simulink model "VSC_GFo_Variable_Frequency_v1"  (R2019b)
settings: Solver=ode1  StartTime=0.0  StopTime=8  FixedStep=Time_Step  MaxStep=1e-5  RelTol=1e-3
undefined symbols (not defined in the file): fb, fn, GRD00_H, GRD00_Lg, GRD00_R, GRD00_Rg, GRD00_TD, GRD00_TN, GRD00_Ub, Time_Step, VSC01_id0, VSC01_Lt_pu, VSC01_mp1, VSC01_mp2, VSC01_mp3, VSC01_Pn, VSC01_R, VSC01_Rt_pu, VSC01_Rv, VSC01_Sn, VSC01_T1, VSC01_T2, VSC01_Tr_PLL, VSC01_Udc_n, VSC01_Udcb, VSC01_Un1, VSC01_Un2, VSC01_W_LF, VSC01_wc1, VSC01_wc2, VSC01_wc3
libraries: powerlib x24, powerlib_meascontrol x1
(part 1 of 2)
settings Model: Creator=Frederic_Colas  LastModifiedBy=xguillau
settings DataIOCC: ReturnWorkspaceOutputs=off
settings OptimizationCC: LifeSpan=inf
settings DebuggingCC: UnconnectedInputMsg=none  UnconnectedOutputMsg=none  UnconnectedLineMsg=none  SFExecutionAtInitializationDiag=none  ArithmeticOperatorsInVariantConditions=warning
settings HardwareCC: ProdBitPerSizeT=32  ProdBitPerPtrDiffT=32  ProdWordSize=32  ProdHWDeviceType=Specified
settings SFSimCC: SimUseLocalCustomCode=off  CustomCodeUndefinedFunction=UseInterfaceOnly
settings RTWCC: RTWUseLocalCustomCode=off
settings CodeAppCC: StateflowObjectComments=on
settings SimscapeCC: SimscapeNormalizeSystem=off

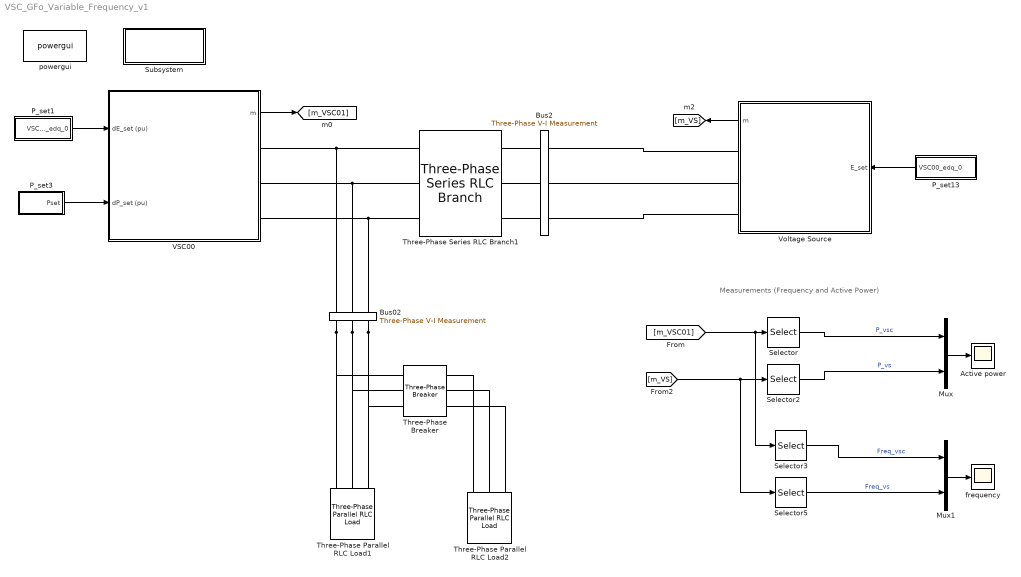
== system VSC_GFo_Variable_Frequency_v1 ==
  note: Measurements (Frequency and Active Power)
  Active power : Scope
  "Bus02 " : powerlib/Measurements/Three-Phase V-I Measurement  VoltageMeasurement=no  SetLabelV=off  LabelV=Vabc  Vpu=off  VpuLL=off  CurrentMeasurement=no  SetLabelI=off  LabelI=Iabc  Ipu=off  Pbase=100e6  Vbase=500e3  OutputType=Complex  PhasorSimulation=off  PSBequivalent=0
      settings: SourceProductName=Simscape Electrical
  Bus2 : powerlib/Measurements/Three-Phase V-I Measurement  VoltageMeasurement=no  SetLabelV=off  LabelV=Vabc  Vpu=off  VpuLL=off  CurrentMeasurement=no  SetLabelI=off  LabelI=Iabc  Ipu=off  Pbase=1e9  Vbase=VSC01_Un2  OutputType=Complex  PhasorSimulation=off  PSBequivalent=0
      settings: SourceProductName=Simscape Electrical
  Mux : Mux  Inputs=2
  Mux1 : Mux  Inputs=2
  P_set1 : Subsystem
  P_set13 : Subsystem
  P_set3 : Subsystem
  Selector : Selector  InputPortWidth=3  IndexOptions=Index vector (dialog)  Indices=[1]  OutputSizes=1
  Selector2 : Selector  InputPortWidth=2  IndexOptions=Index vector (dialog)  Indices=[1]  OutputSizes=1
  Selector3 : Selector  InputPortWidth=3  IndexOptions=Index vector (dialog)  Indices=3  OutputSizes=1
  Selector5 : Selector  InputPortWidth=2  IndexOptions=Index vector (dialog)  Indices=2  OutputSizes=1
  Subsystem : Subsystem
      settings: OpenFcn=LoadFlow_VSC
      mask Display: color('blue'),disp('Update Loadflow')
  Three-Phase Parallel RLC Load1 : powerlib/Elements/Three-Phase Parallel RLC Load  LConnTagsString=A|B|C  Configuration=Y (grounded)  NominalVoltage=GRD00_Un  Vabc=[1e3 1e3 1e3]  Vabcp=[1e3 1e3 1e3]  NominalFrequency=fb  UnbalancedPower=off  ActivePower=100e6  InductivePower=0  CapacitivePower=0  Pabc=[10e3 9e3 11e3]  QLabc=[100 90 110]  QCabc=[100 90 110]  Pabcp=[10e3 9e3 11e3]  QLabcp=[100 90 110]  QCabcp=[100 90 110]  Measurements=None  LoadType=constant Z
      settings: SourceProductName=Simscape Electrical
  Three-Phase Parallel RLC Load2 : powerlib/Elements/Three-Phase Parallel RLC Load  LConnTagsString=A|B|C  Configuration=Y (grounded)  NominalVoltage=GRD00_Un  Vabc=[1e3 1e3 1e3]  Vabcp=[1e3 1e3 1e3]  NominalFrequency=fb  UnbalancedPower=off  ActivePower=400e6  InductivePower=0  CapacitivePower=0  Pabc=[10e3 9e3 11e3]  QLabc=[100 90 110]  QCabc=[100 90 110]  Pabcp=[10e3 9e3 11e3]  QLabcp=[100 90 110]  QCabcp=[100 90 110]  Measurements=None  LoadType=constant Z
      settings: SourceProductName=Simscape Electrical
  Three-Phase Series RLC Branch1 : powerlib/Elements/Three-Phase Series RLC Branch  LConnTagsString=A|B|C  RConnTagsString=A|B|C  BranchType=RL  Resistance=GRD00_Rg  Inductance=GRD00_Lg  Capacitance=1e-6  Measurements=None
      settings: SourceProductName=Simscape Electrical
  Three-Phase Breaker : powerlib/Elements/Three-Phase Breaker  InitialState=open  SwitchA=on  SwitchB=on  SwitchC=on  SwitchTimes=[1 60]  External=off  BreakerResistance=0.01  SnubberResistance=1e6  SnubberCapacitance=inf  Measurements=None
      settings: SourceProductName=Simscape Electrical
  VSC00 : Subsystem  mask(VSC){fb=fb, Sn=VSC01_Sn, Pn=VSC01_Pn, Un1=VSC01_Un1, Un2=VSC01_Un2, Rt_pu=VSC01_Rt_pu, Lt_pu=VSC01_Lt_pu, Lm_pu=500, Rm_pu=500, Tr_PLL=VSC01_Tr_PLL, Val_Freq_Support=on, R_percent=VSC01_R, Rv=VSC01_Rv, W_TVR=VSC01_W_LF, gainpopup=1, wc1=VSC01_wc1, mp1=VSC01_mp1, wc2=VSC01_wc2, mp2=VSC01_mp2, wc3=VSC01_wc3, mp3=VSC01_mp3, T1=VSC01_T1, T2=VSC01_T2, LFpopup=PQ, P0=0.05, Q0=1.0092e-06, V0=1, Theta0=-0.14359}
      mask prompts: fb "Nominal Frequency (Hz)"; Sn "Nominal Apparent Power (VA)"; Pn "Nominal Power (W)"; Un1 "VSC side Nominal Ph-Ph Voltage (V)"; Un2 "Grid side Nominal Ph-Ph Voltage (V)"; Rt_pu "R (pu)"; Lt_pu "L (pu)"; Lm_pu "Rm (pu)"; Rm_pu "Lm (pu)"; Tr_PLL "Time response (s)"; Val_Freq_Support "Frequency Support"; R_percent "Droop Gain (%)"; Rv "Damping Resistance (Rv)"; W_TVR "Dr filter"; gainpopup "Strategy"; wc1 "wc"; mp1 "mp"; wc2 "wc"; mp2 "mp"; wc3 "wc"; mp3 "mp"; P0 "Initial Active Power (pu)"; Q0 "Initial Reactive Power (pu)"; V0 "Initial Voltage (pu)"; Theta0 "Initial Angle (°)"
      mask init:
      | % Update Name of LF bus for internal purpose
      |     NameStr = [get_param(gcb,'Name')];% '_LF'];
      |     set_param([gcb '/Load Flow Bus'],'ID',NameStr);
      |     %disp(NameStr);
      |     
      | % Increase size of Mask dialog box
      |    % pause(0.1);
      |     
      |     
      | % Base values
      |     %Un = Un1;
      |     Pb = Pn;
      |     cos_phi_n = Pn/Sn;
      |     Sb = Pb/cos_phi_n;
      |     %Ub = Un;
      |     Vn = Un1/sqrt(3);
      |     Vb = Vn;
      |     %Ib = Sb / Ub;
      |     Ib = Sb / (3*Vb);
      |     wb = 2*pi*fb;
      |   
      | % PLL derivation of the parameters
      |     wn_PLL=5/Tr_PLL;
      |     zeta_PLL = 1;
      |     Kp_PLL_pu = 2*zeta_PLL*wn_PLL/wb;
      |     Ki_PLL_pu = wn_PLL^2/wb;
      |     
      | % Set the chosen strategy
      |     Chosen_Strategy = str2double(gainpopup);
      |     
      | % Set the frequency droop gain
      |     R = R_percent;
      | 
      | % Compute Initial Voltage of VSC 
      | %   from steady-state output transformer model and Loadflow result
      |     if (LFpopup == 'PQ')
      |         V0 = 1;
      |     end
      |         
      |     R1_pu = Rt_pu/2;
      |     L1_pu = Lt_pu/2;
      |     R2_pu = Rt_pu/2;
      |     L2_pu = Lt_pu/2;
      |     X1_pu = L1_pu;
      |     X2_pu = L2_pu;
      |     Xm_pu = Lm_pu;
      |     
      |     Zm_pu = 1/(1/Rm_pu+1/(1i*Xm_pu));
      | 
      |     S0=P0+1i*Q0;
      |     I2 = conj(S0)/(V0);
      | 
      |     Vm = (R2_pu+1i*X2_pu)*I2 + V0;
      |     Im = Vm/Zm_pu;
      | 
      |     I1 = I2 + Im;
      |     V1 = (R1_pu+1i*X1_pu) * I1 + Vm;
      | 
      |     Vvsc0 = abs(V1);
      |    % disp(Vvsc0*1000)
      |     Theta_vsc0 = angle(V1) * 180/pi+Theta0;
      |     
      |     %vd0=Vvsc0*cos(Theta0*2*pi/180);
      |     %vq0=Vvsc0*sin(Theta0*2*pi/180); 
      |  
      |     %Va0 = Vvsc0*sqrt(2)*Ub/sqrt(3)*sin(Theta_vsc0*pi/180);
      |     %Vb0 = Vvsc0*sqrt(2)*Ub/sqrt(3)*sin(Theta_vsc0*pi/180-2*pi/3);
      |     %Vc0 = Vvsc0*sqrt(2)*Ub/sqrt(3)*sin(Theta_vsc0*pi/180+2*pi/3);
      |     
      |     Va0 = Vvsc0*sqrt(2)*Vb*sin(Theta_vsc0*pi/180);
      |     Vb0 = Vvsc0*sqrt(2)*Vb*sin(Theta_vsc0*pi/180-2*pi/3);
      |     Vc0 = Vvsc0*sqrt(2)*Vb*sin(Theta_vsc0*pi/180+2*pi/3);
      |     
      | % Generate string to display LF results on Mask
      |     %str_tmp = fprintf("Vvsc0 = %d, Theta_vsc0 = %d°",Vvsc0,Theta_vsc0);
      |     mo = get_param(gcb,'MaskObject');
      |     mo.getDialogControl('LF_vsc_str').Prompt = ['V0 = ', num2str(Vvsc0),' pu, Angle = ', num2str(Theta_vsc0),'°'];
      |     mo.getDialogControl('LF_pcc_str').Prompt = ['V0 = ', num2str(V0),' pu, Angle = ', num2str(Theta0),'°'];
      |     mo.getDialogControl('LF_pcc_Power_str').Prompt = ['P0 = ', num2str(P0),' pu, Q0 = ', num2str(Q0),' pu'];
      |     %set_param([gcb],'LF_str',str_tmp);
      |  %GRD00_Theta0 = Theta0;
      |  %P0 = 200e6;
      |  %Q0 = 0;
      |  % Initial current values of VSC (dq pu) 
      |  %id0 =(P0*vd0+Q0*vq0)/(vd0^2+vq0^2) * 1/Ib; %
      |  %iq0 =(P0*vq0-Q0*vd0)/(vd0^2+vq0^2) * 1/Ib; %Initial current in the connexion inductance
      settings: OpenFcn=|
      | NameStr = get_param(gcb,'Name');
      | open_system(gcbh, 'Mask');
      | 
      | h2AllOpenDlgs = DAStudio.ToolRoot.getOpenDialogs;
      | 
      | for i=1:length(h2AllOpenDlgs)
      |     try
      |          %disp(h2AllOpenDlgs(i).getSource.getBlock.Name);
      |         Dialog_block_name = h2AllOpenDlgs(i).getSource.getBlock.Name;
      |          %strcmp(Dialog_block_name, NameStr),
      |         if (strcmp(h2AllOpenDlgs(i).getSource.getBlock.Name, NameStr))
      |             iPos = h2AllOpenDlgs(i).position;
      |             h2AllOpenDlgs(i).position = [iPos(1)   iPos(2)   iPos(3)*1.4   iPos(4)];
      |         end
      |     end
      | end
      mask TypeOptions gainpopup: 1 | 2 | 3
      mask Callback gainpopup:
      | % Get the mask parameter values. This is a cell
      | %   array of character vectors.
      | maskStr = get_param(gcb,'gainpopup');
      | p=Simulink.Mask.get(gcb);
      | 
      | % The pop-up menu is the first mask parameter.
      | %   Check the value selected in the pop-up
      | if strcmp(maskStr,'1'),
      | 
      |     % Set the visibility of both parameters on when
      |     %   User-defined is selected in the pop-up.
      |     p.getDialogControl('Param_Strat_1').Visible='on';
      |     p.getDialogControl('Param_Strat_2').Visible='off';
      |     p.getDialogControl('Param_Strat_3').Visible='off';
      | 
      | elseif strcmp(maskStr,'2'),
      | 
      |     % Set the visibility of both parameters on when
      |     %   User-defined is selected in the pop-up.
      |     p.getDialogControl('Param_Strat_1').Visible='off';
      |     p.getDialogControl('Param_Strat_2').Visible='on';
      |     p.getDialogControl('Param_Strat_3').Visible='off';
      | 
      |     % Turn off the visibility of the Value field
      |     %   when User-defined is not selected.
      | else
      | 
      |     % Set the visibility of both parameters on when
      |     %   User-defined is selected in the pop-up.
      |     p.getDialogControl('Param_Strat_1').Visible='off';
      |     p.getDialogControl('Param_Strat_2').Visible='off';
      |     p.getDialogControl('Param_Strat_3').Visible='on';
      | 
      | end
      mask TypeOptions LFpopup: Swing | PQ | PV
      mask Callback LFpopup:
      | % Get the mask parameter values. This is a cell
      | %   array of character vectors.
      | maskStr = get_param(gcb,'LFpopup');
      | p=Simulink.Mask.get(gcb);
      | 
      | % The pop-up menu is the first mask parameter.
      | %   Check the value selected in the pop-up
      | if strcmp(maskStr,'Swing'),
      | 
      |     % Set the visibility of both parameters on when
      |     %   User-defined is selected in the pop-up.
      |     p.getParameter('P0').Visible='off';
      |     p.getParameter('Q0').Visible='off';
      |     p.getParameter('V0').Visible='on';
      |     p.getParameter('Theta0').Visible='on';
      |     set_param([gcb '/Source_For_LF'],'BusType','swing');
      | 
      | elseif strcmp(maskStr,'PQ'),
      | 
      |     % Set the visibility of both parameters on when
      |     %   User-defined is selected in the pop-up.
      |     p.getParameter('P0').Visible='on';
      |     p.getParameter('Q0').Visible='on';
      |     p.getParameter('V0').Value='1';
      |     set_param(gcb,'V0','1');
      |     p.getParameter('V0').Visible='off';
      |     p.getParameter('Theta0').Visible='off';
      |     set_param([gcb '/Source_For_LF'],'BusType','PQ');
      | 
      |     % Turn off the visibility of the Value field
      |     %   when User-defined is not selected.
      | else
      | 
      |     % Set the visibility of both parameters on when
      |     %   User-defined is selected in the pop-up.
      |     p.getParameter('P0').Visible='on';
      |     p.getParameter('Q0').Visible='off';
      |     p.getParameter('V0').Visible='on';
      |     p.getParameter('Theta0').Visible='off';
      |     set_param([gcb '/Source_For_LF'],'BusType','PV');
      | 
      | end
      mask DialogControl Nominal_Param Prompt: Nominal Value
      mask DialogControl Container20 Prompt: Output Transformer
      mask DialogControl Control_Param Prompt: Control Parameter
      mask DialogControl Container13 Prompt: PLL
      mask DialogControl Container14 Prompt: Frequency Support
      mask DialogControl Container15 Prompt: Transient Virtual Resistor
      mask DialogControl Container18 Prompt: Control Strategy
      mask DialogControl Title_Strat_1 Prompt: Strategy 1
      mask DialogControl Title_Strat_2 Prompt: Strategy 2
      mask DialogControl Title_Strat_3 Prompt: Strategy 3
      mask DialogControl LF_Param Prompt: Loadflow
      mask DialogControl Control4 Prompt: Initial Operating Point
      mask DialogControl Container24 Prompt: VSC side
      mask DialogControl LF_vsc_str Prompt: V0 = 1.0004 pu, Angle = 0.29428°
      mask DialogControl Container25 Prompt: PCC
      mask DialogControl LF_pcc_str Prompt: V0 = 1 pu, Angle = -0.14359°
      mask DialogControl LF_pcc_Power_str Prompt: P0 = 0.05 pu, Q0 = 1.0092e-06 pu
      mask DialogControl UpdateLoadflow Prompt: Update Loadflow
      mask DialogControl UpdateLoadflow Callback: Load_Flow_VSC
  Voltage Source : Subsystem  mask(Inertial_Voltage_source){fb=fb, Sc=1e9, Ub=GRD00_Ub, H_eq=GRD00_H, Droop=GRD00_R, TN=GRD00_TN, TD=GRD00_TD, P0=0.050122}
      mask prompts: fb "Nominal Frequency (Hz)"; Sc "Nominal Power (VA)"; Ub "Nominal Voltage (V)"; H_eq "Inertial Constant H (s)"; Droop "Droop Gain"; TN "Lead Time Constant"; TD "Lag Time Constant"; P0 "Initial Power"
      mask init:
      | % Update Name of LF bus for internal purpose
      |     NameStr = [get_param(gcb,'Name')];% '_LF'];
      |     set_param([gcb '/Load Flow Bus'],'ID',NameStr);
      | 
      | % Base values
      |     wb=2*pi*fb;
      |     Ib=Sc/(sqrt(3)*Ub);
      |     Vb=Ub/sqrt(3);
      |     e0=Vb;
      |     Theta_e0=0;
      |     P0_VS = P0;
      |   
      | % Parameters
      |     R=Droop;
      mask DialogControl Container5 Prompt: Nominal Values
      mask DialogControl Container16 Prompt: Network Time Constants
  frequency : Scope
  powergui : powerlib/powergui  Priority=1  SimulationMode=Discrete  SampleTime=Time_Step  frequency=60  Iterations=50  frequencyindice=50  Pbase=1000e6  ErrMax=1e-4  UnitsV=kV  UnitsW=MW  buscounter=0  FunctionMessages=off  echomessages=off  EnableUseOfTLC=off  CurrentSourceSwitches=off  DisableSnubberDevices=off  DisableRonSwitches=off  DisableVfSwitches=off  DisplayEquations=off  AutomaticDiscreteSolvers=off  SolverType=Tustin/Backward Euler (TBE)  Interpol=off  ExternalGateDelay=off  methode=off  Ts=100  x0status=blocks  SPID=on  SwTol=0  HookPort=off  NonlinearTolerance=1e-4  nMaxIteration=100  ContinueOnMaxIteration=off  RestoreLinks=warning  ResistiveCurrentMeasurement=off  Frange=[0:2:500]  Ylog=off  Xlog=on  ShowGrid=off  save=off  variable=ZData  structure=0  ZoomFFT=off  StartTime=0.0  cycles=1  DisplayStyle=1  fundamental=60  FreqAxis=off  MaxFrequency=1000  frequencyindicesteady=1  RmsSteady=1  display=off
      settings: SourceProductName=Simscape Electrical
  wires:
  VSC00/1(m) -> [m_VSC01]
  P_set1/1(VSC01_edq_0) -> VSC00/1(dE_set (pu))
  P_set3/1(Pset) -> VSC00/2(dP_set (pu))
  Voltage Source/1("m ") -> [m_VS]
  P_set13/1(VSC00_edq_0) -> Voltage Source/1(E_set)
  Mux1/1 -> frequency/1
  [m_VS] -> Selector5/1, Selector2/1
  [m_VSC01] -> Selector3/1, Selector/1
  Selector5/1 -> Mux1/2  "Freq_vs"
  Mux/1 -> Active power/1
  Selector2/1 -> Mux/2  "P_vs"
  Selector3/1 -> Mux1/1  "Freq_vsc"
  Selector/1 -> Mux/1  "P_vsc"
  connections:
  Three-Phase Series RLC Branch1/LConn1 -- "Bus02 "/LConn3 -- VSC00/RConn1
  Three-Phase Series RLC Branch1/RConn2 -- Bus2/LConn2
  Three-Phase Series RLC Branch1/LConn3 -- "Bus02 "/LConn1 -- VSC00/RConn3
  Three-Phase Series RLC Branch1/LConn2 -- "Bus02 "/LConn2 -- VSC00/RConn2
  Three-Phase Series RLC Branch1/RConn3 -- Bus2/LConn3
  Three-Phase Series RLC Branch1/RConn1 -- Bus2/LConn1
  Voltage Source/RConn1 -- Bus2/RConn1
  Voltage Source/RConn2 -- Bus2/RConn2
  Voltage Source/RConn3 -- Bus2/RConn3
  "Bus02 "/RConn1 -- Three-Phase Breaker/LConn3 -- Three-Phase Parallel RLC Load1/LConn3
  "Bus02 "/RConn3 -- Three-Phase Breaker/LConn1 -- Three-Phase Parallel RLC Load1/LConn1
  "Bus02 "/RConn2 -- Three-Phase Breaker/LConn2 -- Three-Phase Parallel RLC Load1/LConn2
  Three-Phase Breaker/RConn1 -- Three-Phase Parallel RLC Load2/LConn1
  Three-Phase Parallel RLC Load2/LConn3 -- Three-Phase Breaker/RConn3
  Three-Phase Parallel RLC Load2/LConn2 -- Three-Phase Breaker/RConn2

== system VSC_GFo_Variable_Frequency_v1/P_set1 ==
  Mux : Mux  Inputs=2
  ed0 : Constant  Value=0
  eq0 : Constant  Value=0
  VSC01_edq_0 : Outport  VectorParamsAs1DForOutWhenUnconnected=off
  wires:
  eq0/1 -> Mux/2
  ed0/1 -> Mux/1
  Mux/1 -> VSC01_edq_0/1

== system VSC_GFo_Variable_Frequency_v1/P_set13 ==
  Mux : Mux  Inputs=2
  ed1 : Constant  Value=0
  eq1 : Constant
  VSC00_edq_0 : Outport  VectorParamsAs1DForOutWhenUnconnected=off
  wires:
  Mux/1 -> VSC00_edq_0/1
  eq1/1 -> Mux/1
  ed1/1 -> Mux/2

== system VSC_GFo_Variable_Frequency_v1/P_set3 ==
  D_Pset : Step  Time=0  After=0  SampleTime=0
  P_set : Constant  Value=0
  Sum9 : Sum  Inputs=++|
  Pset : Outport  VectorParamsAs1DForOutWhenUnconnected=off
  wires:
  D_Pset/1 -> Sum9/1
  Sum9/1 -> Pset/1
  P_set/1 -> Sum9/2

== system VSC_GFo_Variable_Frequency_v1/Subsystem ==

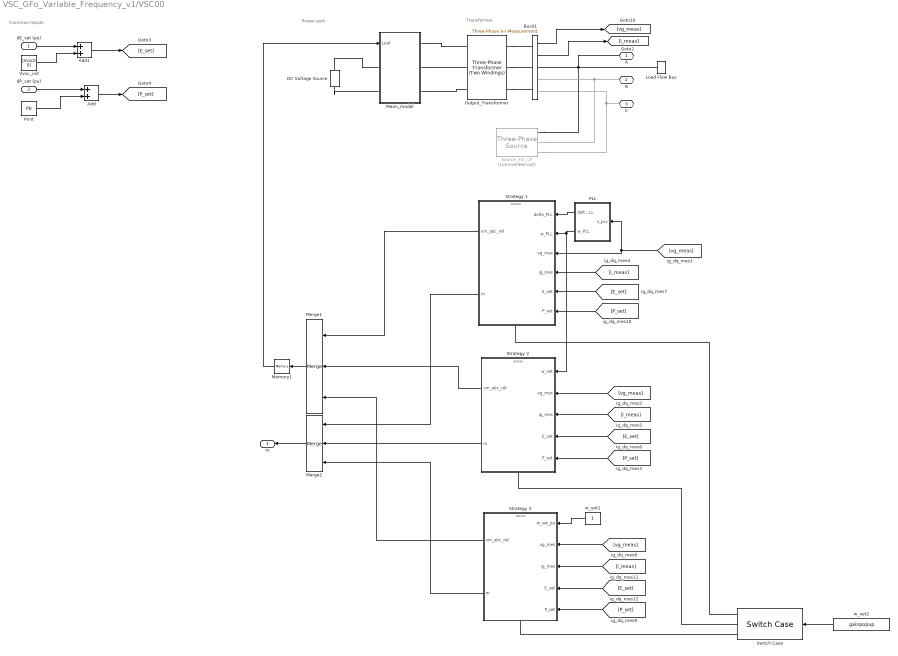
== system VSC_GFo_Variable_Frequency_v1/VSC00 ==
  note: Power part
  note: Common Inputs
  note: Transformer
  dE_set (pu) : Inport
  dP_set (pu) : Inport  Port=2
  Add : Sum
  Add1 : Sum
  Bus01 : powerlib/Measurements/Three-Phase V-I Measurement  VoltageMeasurement=phase-to-ground  SetLabelV=off  LabelV=Vabc  Vpu=off  VpuLL=off  CurrentMeasurement=yes  SetLabelI=off  LabelI=Iabc  Ipu=off  Pbase=100e6  Vbase=500e3  OutputType=Complex  PhasorSimulation=off  PSBequivalent=0
      settings: SourceProductName=Simscape Electrical
  DC Voltage Source : powerlib/Electrical Sources/DC Voltage Source  Amplitude=VSC01_Udc_n  Measurements=Voltage
      settings: SourceProductName=Simscape Electrical
  Load Flow Bus : powerlib/Measurements/Load Flow Bus  LConnTagsString=a  Phases=single  Connectors=on one side  ID=VSC00  Vbase=Un2  Vref=V0  Vangle=Theta0  VLF=0.9997  VLFb=1  VLFc=1  angleLF=-0.1436  angleLFb=0  angleLFc=0
      settings: SourceProductName=Simscape Electrical
  Mean_model : Subsystem
  Memory1 : Memory  InitialCondition=[Va0 Vb0 Vc0]
  Merge1 : Merge  Inputs=3
  Merge2 : Merge  Inputs=3
  Output_Transformer : powerlib/Elements/Three-Phase Transformer (Two Windings)  Winding1Connection=Yg  Winding2Connection=Yg  CoreType=Three single-phase transformers  SetSaturation=off  Hysteresis=off  DataFile='hysteresis'  SetInitialFlux=off  Measurements=None  UNITS=pu  NominalPower=[Sn , fn ]  Winding1=[Un1 , Rt_pu/2 , Lt_pu/2]  Winding2=[Un2 , Rt_pu/2 , Lt_pu/2]  Rm=Rm_pu  Lm=Lm_pu  L0=0.5  Saturation=[ 0,0 ; 0.0024,1.2 ; 1.0,1.52 ]  InitialFluxes=[ 0.8 , -0.8 , 0.7 ]  BreakLoop=off  DiscreteSolver=Trapezoidal iterative  DataType=off  TransfoNumber=1
      settings: SourceProductName=Simscape Electrical
  PLL : Subsystem
  Pinit : Constant  Value=P0
  Source_For_LF : powerlib/Electrical Sources/Three-Phase Source  Commented=on  InternalConnection=Yg  VoltagePhases=off  Voltage=(400000)*0.999746  PhaseAngle=-0.14359  Voltage_phases=[25e3 25e3 25e3]/sqrt(3)  PhaseAngles_phases=[0 -120 +120]  Frequency=50  NonIdealSource=off  SpecifyImpedance=off  Resistance=0  Inductance=0  ShortCircuitLevel=100e6  BaseVoltage=Un  XRratio=7  BusType=PQ  Pref=P0*Sb  Qref=Q0*Sb  Prefabc=[10e3, 10e3, 10e3]  Qrefabc=[0, 0, 0]  Qmin=-inf  Qmax=inf
      settings: SourceProductName=Simscape Electrical
  Strategy 1 : Subsystem
  Strategy 2 : Subsystem
  Strategy 3 : Subsystem
  Switch Case : SwitchCase  CaseConditions={1,2,3}  ShowDefaultCase=off
  Vvsc_init : Constant  Value=[Vvsc0 0]
  w_set1 : Constant
  w_set2 : Constant  Value=gainpopup
  A : PMIOPort  Side=Right
  B : PMIOPort  Port=2  Side=Right
  C : PMIOPort  Port=3  Side=Right
  m : Outport  VectorParamsAs1DForOutWhenUnconnected=off
  wires:
  PLL/1(delta_PLL) -> Strategy 1/1(delta_PLL)
  w_set1/1 -> Strategy 3/1(w_set_pu)
  Add/1 -> [P_set]
  [i_meas] -> Strategy 2/3(ig_mes)
  Strategy 2/2(m) -> Merge2/2
  [i_meas] -> Strategy 1/4(ig_mes)
  Switch Case/1 -> Strategy 1/Action
  [vg_meas] -> Strategy 3/2(vg_mes)
  [vg_meas] -> PLL/1(v_pcc), Strategy 1/3(vg_mes)
  [E_set] -> Strategy 2/4(E_set)
  Merge2/1 -> m/1
  Bus01/2 -> [i_meas]
  dE_set (pu)/1 -> Add1/1
  Strategy 1/1(vm_abc_ref) -> Merge1/1
  [i_meas] -> Strategy 3/3(ig_mes)
  Switch Case/3 -> Strategy 3/Action
  [E_set] -> Strategy 3/4(E_set)
  Strategy 1/2(m) -> Merge2/1
  w_set2/1 -> Switch Case/1
  Bus01/1 -> [vg_meas]
  [P_set] -> Strategy 3/5(P_set)
  Strategy 3/2(m) -> Merge2/3
  PLL/2(w_PLL) -> Strategy 1/2(w_PLL), Strategy 2/1(w_set)
  Add1/1 -> [E_set]
  [P_set] -> Strategy 2/5(P_set)
  Strategy 2/1(vm_abc_ref) -> Merge1/2
  Vvsc_init/1 -> Add1/2
  Merge1/1 -> Memory1/1
  [P_set] -> Strategy 1/6(P_set)
  Strategy 3/1(vm_abc_ref) -> Merge1/3
  Pinit/1 -> Add/2
  Switch Case/2 -> Strategy 2/Action
  dP_set (pu)/1 -> Add/1
  [E_set] -> Strategy 1/5(E_set)
  [vg_meas] -> Strategy 2/2(vg_mes)
  Memory1/1 -> Mean_model/1(Uref)
  connections:
  Source_For_LF/RConn3 -- Bus01/RConn3 -- C/RConn1
  Load Flow Bus/LConn1 -- Source_For_LF/RConn1 -- Bus01/RConn1 -- A/RConn1
  Mean_model/RConn3 -- Output_Transformer/LConn3
  Mean_model/RConn2 -- Output_Transformer/LConn2
  Mean_model/RConn1 -- Output_Transformer/LConn1
  Source_For_LF/RConn2 -- Bus01/RConn2 -- B/RConn1
  Output_Transformer/RConn3 -- Bus01/LConn3
  DC Voltage Source/RConn1 -- Mean_model/LConn1
  Output_Transformer/RConn2 -- Bus01/LConn2
  Output_Transformer/RConn1 -- Bus01/LConn1
  DC Voltage Source/LConn1 -- Mean_model/LConn2

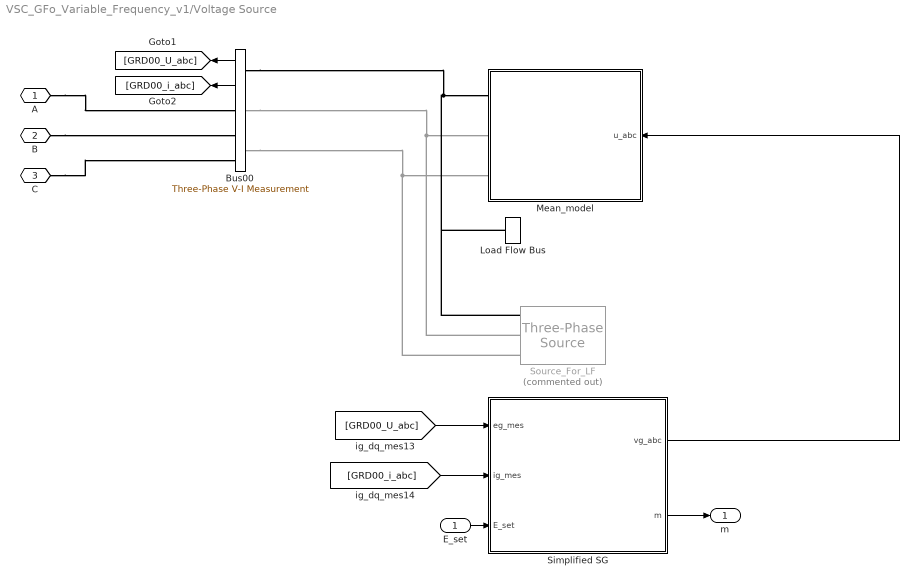
== system VSC_GFo_Variable_Frequency_v1/Voltage Source ==
  E_set : Inport
  Bus00 : powerlib/Measurements/Three-Phase V-I Measurement  VoltageMeasurement=phase-to-ground  SetLabelV=off  LabelV=Vabc  Vpu=off  VpuLL=off  CurrentMeasurement=yes  SetLabelI=off  LabelI=Iabc  Ipu=off  Pbase=100e6  Vbase=500e3  OutputType=Complex  PhasorSimulation=off  PSBequivalent=0
      settings: SourceProductName=Simscape Electrical
  Load Flow Bus : powerlib/Measurements/Load Flow Bus  LConnTagsString=a  Phases=single  Connectors=on one side  ID=Voltage Source  Vbase=Ub  Vref=1  Vangle=0  VLF=1  VLFb=1  VLFc=1  angleLF=0  angleLFb=0  angleLFc=0
      settings: SourceProductName=Simscape Electrical
  Mean_model : Subsystem
  Simplified SG : Subsystem
  Source_For_LF : powerlib/Electrical Sources/Three-Phase Source  Commented=on  InternalConnection=Yg  VoltagePhases=off  Voltage=(400000)*1  PhaseAngle=0  Voltage_phases=[25e3 25e3 25e3]/sqrt(3)  PhaseAngles_phases=[0 -120 +120]  Frequency=fb  NonIdealSource=on  SpecifyImpedance=off  Resistance=0  Inductance=0  ShortCircuitLevel=100e6  BaseVoltage=GRD00_Un  XRratio=7  BusType=swing  Pref=P0  Qref=Q0  Prefabc=[10e3, 10e3, 10e3]  Qrefabc=[0, 0, 0]  Qmin=-inf  Qmax=inf
      settings: SourceProductName=Simscape Electrical
  A : PMIOPort  Side=Right
  B : PMIOPort  Port=2  Side=Right
  C : PMIOPort  Port=3  Side=Right
  "m " : Outport  VectorParamsAs1DForOutWhenUnconnected=off
  wires:
  [GRD00_U_abc] -> Simplified SG/1(eg_mes)
  E_set/1 -> Simplified SG/3(E_set)
  Simplified SG/1(vg_abc) -> Mean_model/1(u_abc)
  [GRD00_i_abc] -> Simplified SG/2(ig_mes)
  Simplified SG/2(m) -> "m "/1
  Bus00/1 -> [GRD00_U_abc]
  Bus00/2 -> [GRD00_i_abc]
  connections:
  Source_For_LF/RConn3 -- Bus00/LConn3 -- Mean_model/RConn3
  Source_For_LF/RConn2 -- Bus00/LConn2 -- Mean_model/RConn2
  Source_For_LF/RConn1 -- Load Flow Bus/LConn1 -- Bus00/LConn1 -- Mean_model/RConn1
  A/RConn1 -- Bus00/RConn1
  B/RConn1 -- Bus00/RConn2
  C/RConn1 -- Bus00/RConn3

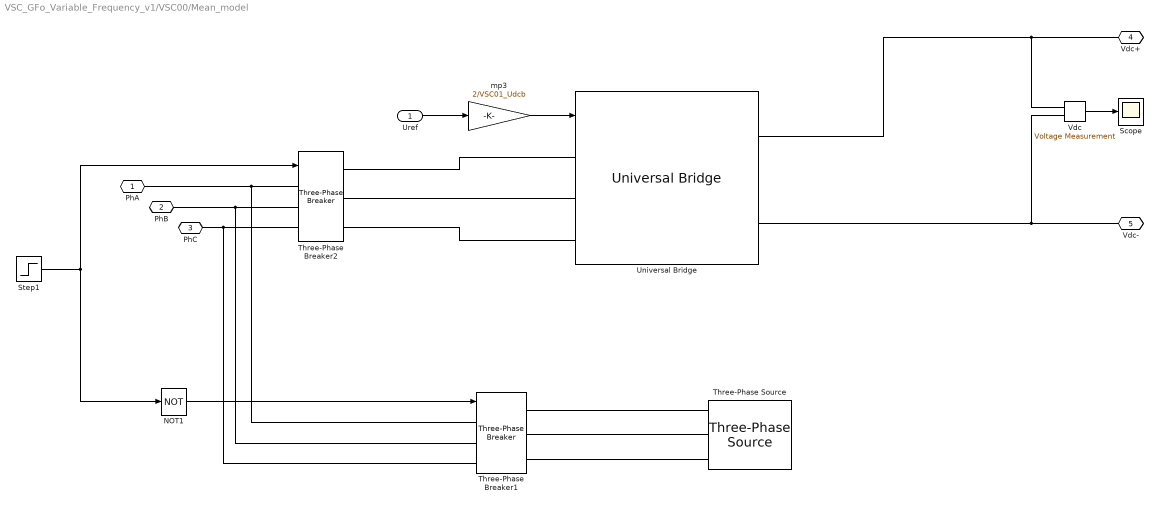
== system VSC_GFo_Variable_Frequency_v1/VSC00/Mean_model ==
  Uref : Inport
  NOT1 : Logic  Operator=NOT  IconShape=distinctive  AllPortsSameDT=off  OutDataTypeStr=boolean
  Scope : Scope
  Step1 : Step  Time=Time_Step  SampleTime=Time_Step
  Three-Phase Breaker1 : powerlib/Elements/Three-Phase Breaker  InitialState=closed  SwitchA=on  SwitchB=on  SwitchC=on  SwitchTimes="[4/60  10/60]"  External=on  BreakerResistance=0.001  SnubberResistance=1e6  SnubberCapacitance=inf  Measurements=None
      settings: SourceProductName=Simscape Electrical
  Three-Phase Breaker2 : powerlib/Elements/Three-Phase Breaker  InitialState=open  SwitchA=on  SwitchB=on  SwitchC=on  SwitchTimes="[4/60  10/60]"  External=on  BreakerResistance=0.001  SnubberResistance=1e6  SnubberCapacitance=inf  Measurements=None
      settings: SourceProductName=Simscape Electrical
  Three-Phase Source : powerlib/Electrical Sources/Three-Phase Source  InternalConnection=Yg  VoltagePhases=off  Voltage=Vvsc0*Un1  PhaseAngle=Theta_vsc0  Voltage_phases=[25e3 25e3 25e3]/sqrt(3)  PhaseAngles_phases=[0 -120 +120]  Frequency=50  NonIdealSource=off  SpecifyImpedance=off  Resistance=0  Inductance=0  ShortCircuitLevel=100e6  BaseVoltage=VSC01_Un1  XRratio=7  BusType=swing  Pref=0.3  Qref=0  Prefabc=[10e3, 10e3, 10e3]  Qrefabc=[0, 0, 0]  Qmin=-Inf  Qmax=Inf
      settings: SourceProductName=Simscape Electrical
  Universal Bridge : powerlib/Power Electronics/Universal Bridge  Arms=3  SnubberResistance=1e5  SnubberCapacitance=inf  Device=Average-model based VSC  Ron=1e-3  Lon=0  ForwardVoltages="[  0  0  ]"  ForwardVoltage=0  GTOparameters=[ 10e-6 , 20e-6 ]  IGBTparameters=[ 1e-6 , 2e-6 ]  Measurements=None  Measurements_2=None  converterType=Rectifier
      settings: SourceProductName=Simscape Electrical
  Vdc : powerlib/Measurements/Voltage Measurement  PhasorSimulation=off  OutputType=Complex  PSBequivalent=0
      settings: SourceProductName=Simscape Electrical
  mp3 : Gain  Gain=2/VSC01_Udcb
  PhA : PMIOPort  Side=Right
  PhB : PMIOPort  Port=2  Side=Right
  PhC : PMIOPort  Port=3  Side=Right
  Vdc+ : PMIOPort  Port=4  Side=Left
  Vdc- : PMIOPort  Port=5  Side=Left
  wires:
  Vdc/1 -> Scope/1
  Uref/1 -> mp3/1
  mp3/1 -> Universal Bridge/1
  Step1/1 -> Three-Phase Breaker2/1, NOT1/1
  NOT1/1 -> Three-Phase Breaker1/1
  connections:
  Vdc-/RConn1 -- Universal Bridge/RConn2 -- Vdc/LConn2
  Vdc+/RConn1 -- Universal Bridge/RConn1 -- Vdc/LConn1
  Three-Phase Source/RConn3 -- Three-Phase Breaker1/RConn3
  Three-Phase Source/RConn2 -- Three-Phase Breaker1/RConn2
  Three-Phase Source/RConn1 -- Three-Phase Breaker1/RConn1
  Three-Phase Breaker2/RConn3 -- Universal Bridge/LConn3
  Three-Phase Breaker2/RConn2 -- Universal Bridge/LConn2
  Three-Phase Breaker2/RConn1 -- Universal Bridge/LConn1
  PhC/RConn1 -- Three-Phase Breaker1/LConn3 -- Three-Phase Breaker2/LConn3
  PhB/RConn1 -- Three-Phase Breaker1/LConn2 -- Three-Phase Breaker2/LConn2
  PhA/RConn1 -- Three-Phase Breaker1/LConn1 -- Three-Phase Breaker2/LConn1

== system VSC_GFo_Variable_Frequency_v1/VSC00/PLL ==
  v_pcc : Inport
  0 - Vd1 : Gain  Gain=1/Vb  SaturateOnIntegerOverflow=on  OutDataTypeStr=Inherit: Same as input  ParamDataTypeStr=Inherit: Same as input
  Correcteur PI : Subsystem
  Scope : Scope
  Terminator : Terminator
  abc --> dq : Subsystem
  delta_PLL : Outport  VectorParamsAs1DForOutWhenUnconnected=off
  w_PLL : Outport  Port=2  VectorParamsAs1DForOutWhenUnconnected=off
  wires:
  v_pcc/1 -> 0 - Vd1/1
  0 - Vd1/1 -> abc --> dq/1(vpcc_abc)
  abc --> dq/2(vpcc_q) -> Scope/1, Correcteur PI/1(In1)
  Correcteur PI/1(w_PLL) -> w_PLL/1
  abc --> dq/1(vpcc_d) -> Terminator/1
  Correcteur PI/2(delta_theta) -> delta_PLL/1, abc --> dq/2(Theta)

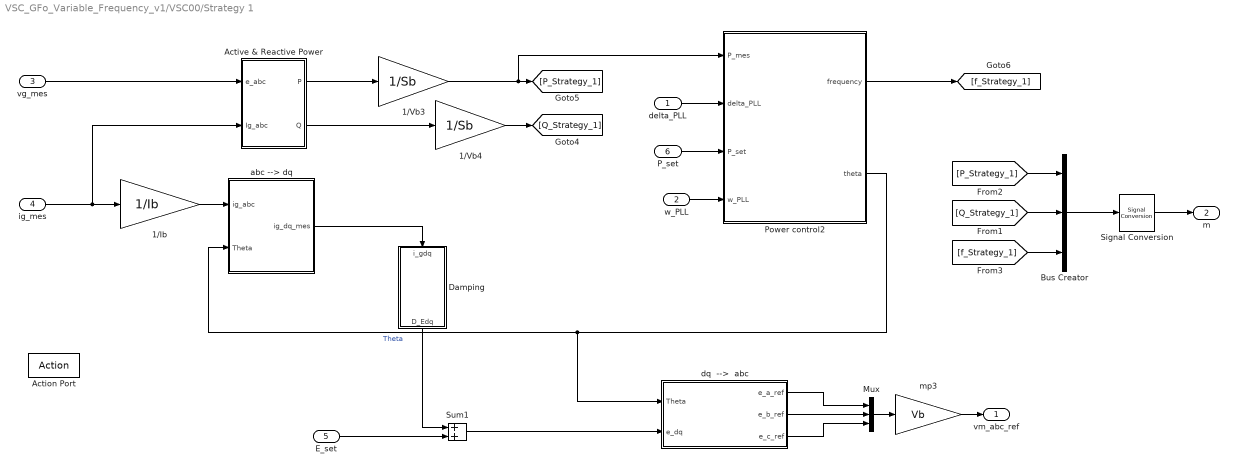
== system VSC_GFo_Variable_Frequency_v1/VSC00/Strategy 1 ==
  delta_PLL : Inport
  w_PLL : Inport  Port=2
  vg_mes : Inport  Port=3
  ig_mes : Inport  Port=4
  E_set : Inport  Port=5
  P_set : Inport  Port=6
  Action Port : ActionPort  ActionPortLabel=case [ 1 ]:
  " Active & Reactive Power" : Subsystem  DialogController=POWERSYS.PowerSysDialog
  1/Ib : Gain  Gain=1/Ib
  1/Vb3 : Gain  Gain=1/Sb
  1/Vb4 : Gain  Gain=1/Sb
  Bus Creator : BusCreator  Inputs=3
  Damping : Subsystem
  Mux : Mux  Inputs=3
  Power control2 : Subsystem
  Signal Conversion : SignalConversion  OverrideOpt=off
  Sum1 : Sum
  abc --> dq : Subsystem
  "dq  -->  abc " : Subsystem
  mp3 : Gain  Gain=Vb
  vm_abc_ref : Outport  VectorParamsAs1DForOutWhenUnconnected=off
  m : Outport  Port=2  VectorParamsAs1DForOutWhenUnconnected=off
  wires:
  Bus Creator/1 -> Signal Conversion/1
  Signal Conversion/1 -> m/1
  [P_Strategy_1] -> Bus Creator/1
  [Q_Strategy_1] -> Bus Creator/2
  [f_Strategy_1] -> Bus Creator/3
  mp3/1 -> vm_abc_ref/1
  1/Ib/1 -> abc --> dq/1(ig_abc)
  "dq  -->  abc "/3(e_c_ref) -> Mux/3
  " Active & Reactive Power"/1(P) -> 1/Vb3/1
  E_set/1 -> Sum1/2
  " Active & Reactive Power"/2(Q) -> 1/Vb4/1
  1/Vb3/1 -> Power control2/1(P_mes), [P_Strategy_1]
  Mux/1 -> mp3/1
  ig_mes/1 -> " Active & Reactive Power"/2(Ig_abc), 1/Ib/1
  1/Vb4/1 -> [Q_Strategy_1]
  "dq  -->  abc "/2(e_b_ref) -> Mux/2
  abc --> dq/1(ig_dq_mes) -> Damping/1(i_gdq)
  "dq  -->  abc "/1(e_a_ref) -> Mux/1
  Sum1/1 -> "dq  -->  abc "/2(e_dq)
  Damping/1("D_Edq ") -> Sum1/1
  delta_PLL/1 -> Power control2/2(delta_PLL)
  P_set/1 -> Power control2/3(P_set)
  w_PLL/1 -> Power control2/4(w_PLL)
  Power control2/1(frequency) -> [f_Strategy_1]
  Power control2/2(theta) -> "dq  -->  abc "/1(Theta), abc --> dq/2(Theta)  "Theta"
  vg_mes/1 -> " Active & Reactive Power"/1(e_abc)

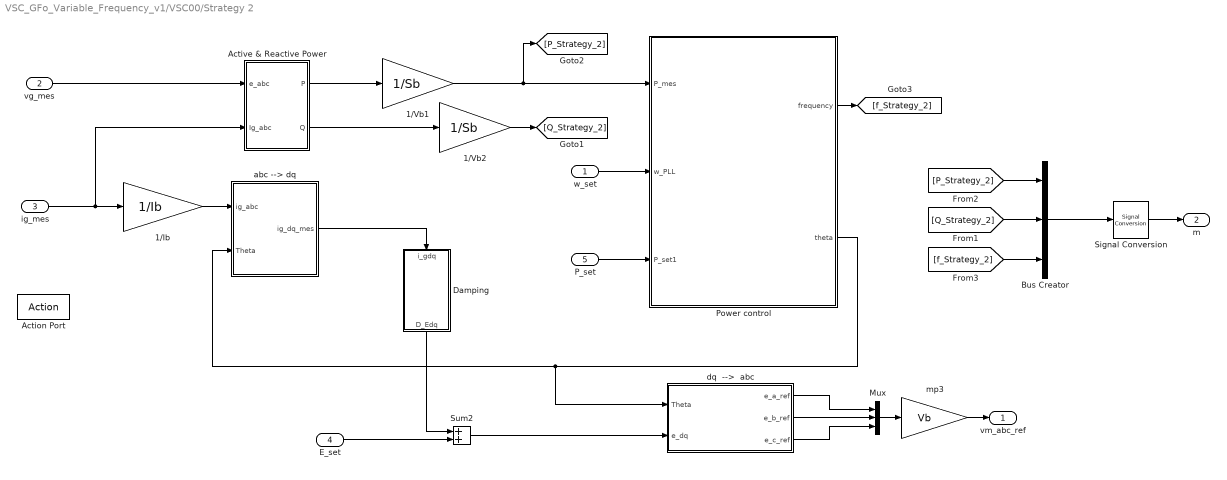
== system VSC_GFo_Variable_Frequency_v1/VSC00/Strategy 2 ==
  w_set : Inport
  vg_mes : Inport  Port=2
  ig_mes : Inport  Port=3
  E_set : Inport  Port=4
  P_set : Inport  Port=5
  Action Port : ActionPort  ActionPortLabel=case [ 2 ]:
  " Active & Reactive Power" : Subsystem  DialogController=POWERSYS.PowerSysDialog
  1/Ib : Gain  Gain=1/Ib
  1/Vb1 : Gain  Gain=1/Sb
  1/Vb2 : Gain  Gain=1/Sb
  Bus Creator : BusCreator  Inputs=3
  Damping : Subsystem
  Mux : Mux  Inputs=3
  Power control : Subsystem
  Signal Conversion : SignalConversion  OverrideOpt=off
  Sum2 : Sum
  abc --> dq : Subsystem
  "dq  -->  abc " : Subsystem
  mp3 : Gain  Gain=Vb
  vm_abc_ref : Outport  VectorParamsAs1DForOutWhenUnconnected=off
  m : Outport  Port=2  VectorParamsAs1DForOutWhenUnconnected=off
  wires:
  w_set/1 -> Power control/2(w_PLL)
  abc --> dq/1(ig_dq_mes) -> Damping/1(i_gdq)
  P_set/1 -> Power control/3(P_set1)
  1/Vb1/1 -> [P_Strategy_2], Power control/1(P_mes)
  1/Vb2/1 -> [Q_Strategy_2]
  E_set/1 -> Sum2/2
  [Q_Strategy_2] -> Bus Creator/2
  Bus Creator/1 -> Signal Conversion/1
  [P_Strategy_2] -> Bus Creator/1
  [f_Strategy_2] -> Bus Creator/3
  Signal Conversion/1 -> m/1
  Power control/1(frequency) -> [f_Strategy_2]
  " Active & Reactive Power"/2(Q) -> 1/Vb2/1
  ig_mes/1 -> " Active & Reactive Power"/2(Ig_abc), 1/Ib/1
  " Active & Reactive Power"/1(P) -> 1/Vb1/1
  vg_mes/1 -> " Active & Reactive Power"/1(e_abc)
  1/Ib/1 -> abc --> dq/1(ig_abc)
  Mux/1 -> mp3/1
  "dq  -->  abc "/1(e_a_ref) -> Mux/1
  mp3/1 -> vm_abc_ref/1
  Power control/2(theta) -> abc --> dq/2(Theta), "dq  -->  abc "/1(Theta)
  "dq  -->  abc "/3(e_c_ref) -> Mux/3
  "dq  -->  abc "/2(e_b_ref) -> Mux/2
  Damping/1("D_Edq ") -> Sum2/1
  Sum2/1 -> "dq  -->  abc "/2(e_dq)

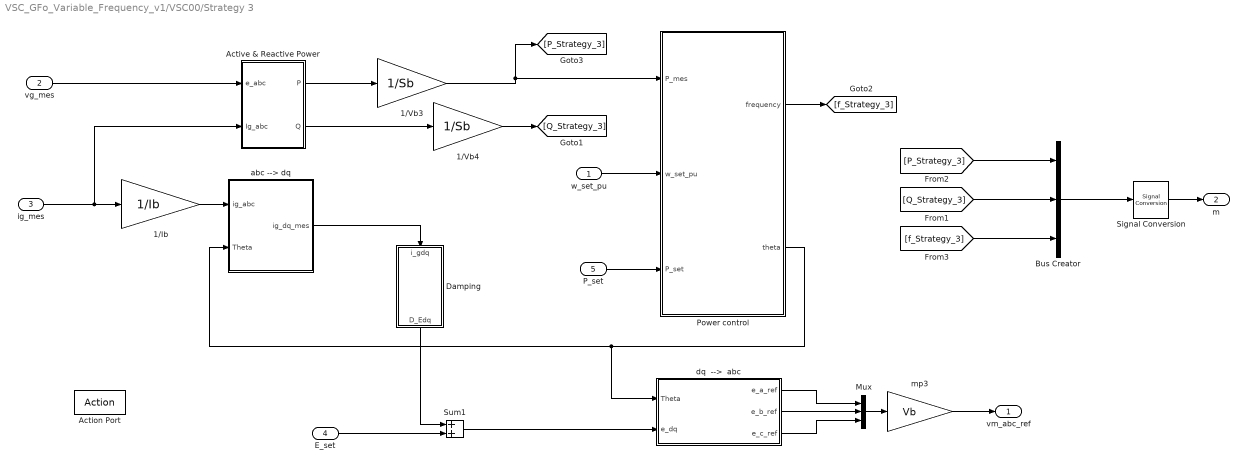
== system VSC_GFo_Variable_Frequency_v1/VSC00/Strategy 3 ==
  w_set_pu : Inport
  vg_mes : Inport  Port=2
  ig_mes : Inport  Port=3
  E_set : Inport  Port=4
  P_set : Inport  Port=5
  Action Port : ActionPort  ActionPortLabel=case [ 3 ]:
  " Active & Reactive Power" : Subsystem  DialogController=POWERSYS.PowerSysDialog
  1/Ib : Gain  Gain=1/Ib
  1/Vb3 : Gain  Gain=1/Sb
  1/Vb4 : Gain  Gain=1/Sb
  Bus Creator : BusCreator  Inputs=3
  Damping : Subsystem
  Mux : Mux  Inputs=3
  Power control : Subsystem
  Signal Conversion : SignalConversion  OverrideOpt=off
  Sum1 : Sum
  abc --> dq : Subsystem
  "dq  -->  abc " : Subsystem
  mp3 : Gain  Gain=Vb
  vm_abc_ref : Outport  VectorParamsAs1DForOutWhenUnconnected=off
  m : Outport  Port=2  VectorParamsAs1DForOutWhenUnconnected=off
  wires:
  Signal Conversion/1 -> m/1
  [Q_Strategy_3] -> Bus Creator/2
  Bus Creator/1 -> Signal Conversion/1
  [P_Strategy_3] -> Bus Creator/1
  [f_Strategy_3] -> Bus Creator/3
  Sum1/1 -> "dq  -->  abc "/2(e_dq)
  "dq  -->  abc "/1(e_a_ref) -> Mux/1
  Damping/1("D_Edq ") -> Sum1/1
  "dq  -->  abc "/2(e_b_ref) -> Mux/2
  1/Vb3/1 -> [P_Strategy_3], Power control/1(P_mes)
  "dq  -->  abc "/3(e_c_ref) -> Mux/3
  " Active & Reactive Power"/2(Q) -> 1/Vb4/1
  ig_mes/1 -> " Active & Reactive Power"/2(Ig_abc), 1/Ib/1
  1/Ib/1 -> abc --> dq/1(ig_abc)
  w_set_pu/1 -> Power control/2(w_set_pu)
  Mux/1 -> mp3/1
  abc --> dq/1(ig_dq_mes) -> Damping/1(i_gdq)
  1/Vb4/1 -> [Q_Strategy_3]
  " Active & Reactive Power"/1(P) -> 1/Vb3/1
  vg_mes/1 -> " Active & Reactive Power"/1(e_abc)
  P_set/1 -> Power control/3(P_set)
  E_set/1 -> Sum1/2
  Power control/1(frequency) -> [f_Strategy_3]
  Power control/2(theta) -> "dq  -->  abc "/1(Theta), abc --> dq/2(Theta)
  mp3/1 -> vm_abc_ref/1

== system VSC_GFo_Variable_Frequency_v1/Voltage Source/Mean_model ==
  u_abc : Inport
  Controlled Voltage Source1 : powerlib/Electrical Sources/Controlled Voltage Source  Initialize=on  Source_Type=AC  Amplitude=e0*sqrt(2)  Phase=0  Frequency=fb  Measurements=None
      settings: SourceProductName=Simscape Electrical
  Controlled Voltage Source2 : powerlib/Electrical Sources/Controlled Voltage Source  Initialize=on  Source_Type=AC  Amplitude=e0*sqrt(2)  Phase=-240  Frequency=fb  Measurements=None
      settings: SourceProductName=Simscape Electrical
  Controlled Voltage Source4 : powerlib/Electrical Sources/Controlled Voltage Source  Initialize=on  Source_Type=AC  Amplitude=e0*sqrt(2)  Phase=-120  Frequency=fb  Measurements=None
      settings: SourceProductName=Simscape Electrical
  Demux : Demux  Outputs=3
  Ground2 : powerlib/Elements/Ground  LConnTagsString=a
      settings: SourceProductName=Simscape Electrical
  A : PMIOPort  Side=Right
  B : PMIOPort  Port=2  Side=Right
  C : PMIOPort  Port=3  Side=Right
  wires:
  u_abc/1 -> Demux/1
  Demux/2 -> Controlled Voltage Source4/1
  Demux/3 -> Controlled Voltage Source2/1
  Demux/1 -> Controlled Voltage Source1/1
  connections:
  Controlled Voltage Source4/LConn1 -- Controlled Voltage Source1/LConn1 -- Controlled Voltage Source2/LConn1 -- Ground2/LConn1
  Controlled Voltage Source2/RConn1 -- C/RConn1
  Controlled Voltage Source4/RConn1 -- B/RConn1
  Controlled Voltage Source1/RConn1 -- A/RConn1

== system VSC_GFo_Variable_Frequency_v1/Voltage Source/Simplified SG ==
  eg_mes : Inport
  ig_mes : Inport  Port=2
  E_set : Inport  Port=3
  " Active & Reactive Power" : Subsystem  DialogController=POWERSYS.PowerSysDialog
  Bus Creator : BusCreator  Inputs=2
  Mux : Mux  Inputs=3
  Power control1 : Subsystem
  Signal Conversion : SignalConversion  OverrideOpt=off
  pu --> SI : Subsystem
  vg_abc : Outport  VectorParamsAs1DForOutWhenUnconnected=off
  m : Outport  Port=2  VectorParamsAs1DForOutWhenUnconnected=off
  wires:
  pu --> SI/1(e_a_SI) -> Mux/1
  ig_mes/1 -> " Active & Reactive Power"/2(Ig_abc)
  eg_mes/1 -> " Active & Reactive Power"/1(e_abc)
  Power control1/3(v_c) -> pu --> SI/3(e_c_pu)
  Mux/1 -> vg_abc/1
  pu --> SI/3(e_c_SI) -> Mux/3
  " Active & Reactive Power"/1(P) -> Power control1/1(P_meas)
  pu --> SI/2(e_b_SI) -> Mux/2
  Power control1/1(v_a) -> pu --> SI/1(e_a_pu)
  Power control1/2(v_b) -> pu --> SI/2(e_b_pu)
  E_set/1 -> Power control1/2(E_set)
  Signal Conversion/1 -> m/1
  Bus Creator/1 -> Signal Conversion/1
  [P_meas] -> Bus Creator/1
  Power control1/4(f_pu) -> Bus Creator/2

== system VSC_GFo_Variable_Frequency_v1/VSC00/PLL/Correcteur PI ==
  In1 : Inport
  0 - Vd1 : Gain  Gain=Kp_PLL_pu  SaturateOnIntegerOverflow=on  OutDataTypeStr=Inherit: Same as input  ParamDataTypeStr=Inherit: Same as input
  0 - Vd2 : Gain  Gain=Ki_PLL_pu  SaturateOnIntegerOverflow=on  OutDataTypeStr=Inherit: Same as input  ParamDataTypeStr=Inherit: Same as input
  Integrator : Integrator
  Integrator1 : Integrator  InitialCondition=Theta0*pi/180
  Sum : Sum  SaturateOnIntegerOverflow=on
  Sum1 : Sum  SaturateOnIntegerOverflow=on
  w_PLL_pu : Gain  Gain=wb  SaturateOnIntegerOverflow=on  OutDataTypeStr=Inherit: Same as input  ParamDataTypeStr=Inherit: Same as input
  w_set : Constant
  w_PLL : Outport  VectorParamsAs1DForOutWhenUnconnected=off
  delta_theta : Outport  Port=2  VectorParamsAs1DForOutWhenUnconnected=off
  wires:
  0 - Vd2/1 -> Integrator/1
  w_set/1 -> Sum1/1
  w_PLL_pu/1 -> Integrator1/1
  Integrator/1 -> Sum/2
  Sum/1 -> Sum1/2
  0 - Vd1/1 -> Sum/1
  In1/1 -> 0 - Vd2/1, 0 - Vd1/1
  Integrator1/1 -> delta_theta/1
  Sum1/1 -> w_PLL/1, w_PLL_pu/1

== system VSC_GFo_Variable_Frequency_v1/VSC00/PLL/abc --> dq ==
  vpcc_abc : Inport
  Theta : Inport  Port=2
  0 - Vd1 : Gain  Gain=1/sqrt(3)  SaturateOnIntegerOverflow=on  OutDataTypeStr=Inherit: Same as input  ParamDataTypeStr=Inherit: Same as input
  abc(SI)->dq (pu) NO FILTER : Subsystem
  vpcc_d : Outport  VectorParamsAs1DForOutWhenUnconnected=off
  vpcc_q : Outport  Port=2  VectorParamsAs1DForOutWhenUnconnected=off
  wires:
  abc(SI)->dq (pu) NO FILTER/2(vpcc_q) -> vpcc_q/1
  vpcc_abc/1 -> 0 - Vd1/1
  Theta/1 -> abc(SI)->dq (pu) NO FILTER/1(Theta)
  abc(SI)->dq (pu) NO FILTER/1(vpcc_d) -> vpcc_d/1
  0 - Vd1/1 -> abc(SI)->dq (pu) NO FILTER/2(e_abc_mes)

== system VSC_GFo_Variable_Frequency_v1/VSC00/Strategy 1/ Active & Reactive Power ==
  e_abc : Inport  PortDimensions=3
  Ig_abc : Inport  Port=2  PortDimensions=3
  Demux : Demux  Outputs=3
  Mux : Mux  Inputs=3
  Product1 : Product  SaturateOnIntegerOverflow=on  InputSameDT=on  OutDataTypeStr=Inherit: Same as first input
  Product3 : Product  SaturateOnIntegerOverflow=on  InputSameDT=on  OutDataTypeStr=Inherit: Same as first input
  Sum : Sum  Inputs=+-  SaturateOnIntegerOverflow=on  InputSameDT=on  OutDataTypeStr=Inherit: Same as first input
  Sum1 : Sum  Inputs=1  SaturateOnIntegerOverflow=on  InputSameDT=on  OutDataTypeStr=Inherit: Same as first input
  Sum4 : Sum  Inputs=1  SaturateOnIntegerOverflow=on  InputSameDT=on  OutDataTypeStr=Inherit: Same as first input
  Sum5 : Sum  Inputs=+-  SaturateOnIntegerOverflow=on  InputSameDT=on  OutDataTypeStr=Inherit: Same as first input
  Sum6 : Sum  Inputs=+-  SaturateOnIntegerOverflow=on  InputSameDT=on  OutDataTypeStr=Inherit: Same as first input
  pu->V : Gain  Gain=1/sqrt(3)  SaturateOnIntegerOverflow=on  OutDataTypeStr=Inherit: Same as input  ParamDataTypeStr=Inherit: Same as input
  P : Outport  VectorParamsAs1DForOutWhenUnconnected=off
  Q : Outport  Port=2  VectorParamsAs1DForOutWhenUnconnected=off
  wires:
  pu->V/1 -> Q/1  "Q"
  Mux/1 -> Product3/1
  Sum6/1 -> Mux/2
  Sum5/1 -> Mux/1
  Sum/1 -> Mux/3
  Demux/3 -> Sum6/1, Sum5/2
  Demux/2 -> Sum5/1, Sum/2
  Demux/1 -> Sum6/2, Sum/1
  Sum4/1 -> P/1  "P"
  Ig_abc/1 -> Product3/2, Product1/2
  e_abc/1 -> Demux/1, Product1/1
  Product1/1 -> Sum4/1
  Product3/1 -> Sum1/1
  Sum1/1 -> pu->V/1

== system VSC_GFo_Variable_Frequency_v1/VSC00/Strategy 1/Damping ==
  i_gdq : Inport
  Filter w_LF : Subsystem
      mask Display: disp('\omega_{LF} / (s + \omega_{LF})','texmode','on')
  Sum5 : Sum  Inputs=|+-
  nq1 : Gain  Gain=Rv
  "D_Edq " : Outport  VectorParamsAs1DForOutWhenUnconnected=off
  wires:
  i_gdq/1 -> nq1/1
  Sum5/1 -> "D_Edq "/1
  Filter w_LF/1(s) -> Sum5/1
  nq1/1 -> Sum5/2, Filter w_LF/1(e)

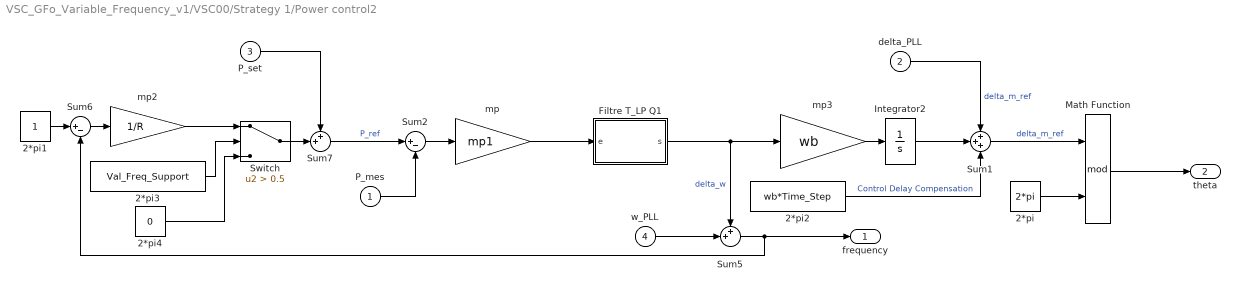
== system VSC_GFo_Variable_Frequency_v1/VSC00/Strategy 1/Power control2 ==
  P_mes : Inport
  delta_PLL : Inport  Port=2
  P_set : Inport  Port=3
  w_PLL : Inport  Port=4
  2*pi : Constant  Value=2*pi
  2*pi1 : Constant
  2*pi2 : Constant  Value=wb*Time_Step
  2*pi3 : Constant  Value=Val_Freq_Support
  2*pi4 : Constant  Value=0
  Filtre T_LP Q1 : Subsystem
  Integrator2 : Integrator  InitialCondition=(Theta_vsc0-Theta0)*pi/180
  Math Function : Math  Operator=mod  SaturateOnIntegerOverflow=on
  Sum1 : Sum  Inputs=+++
  Sum2 : Sum  Inputs=|+-
  Sum5 : Sum  Inputs=++|
  Sum6 : Sum  Inputs=|+-
  Sum7 : Sum  Inputs=++|
  Switch : Switch  Criteria=u2 > Threshold  Threshold=0.5
  mp : Gain  Gain=mp1
  mp2 : Gain  Gain=1/R
  mp3 : Gain  Gain=wb
  frequency : Outport  VectorParamsAs1DForOutWhenUnconnected=off
  theta : Outport  Port=2  VectorParamsAs1DForOutWhenUnconnected=off
  wires:
  Sum2/1 -> mp/1
  Sum1/1 -> Math Function/1  "delta_m_ref"
  2*pi/1 -> Math Function/2
  2*pi1/1 -> Sum6/1
  Sum6/1 -> mp2/1
  P_set/1 -> Sum7/1
  Sum7/1 -> Sum2/1  "P_ref"
  P_mes/1 -> Sum2/2
  Switch/1 -> Sum7/2
  Math Function/1 -> theta/1
  Filtre T_LP Q1/1(s) -> mp3/1, Sum5/1  "delta_w"
  mp3/1 -> Integrator2/1
  mp/1 -> Filtre T_LP Q1/1(e)
  delta_PLL/1 -> Sum1/1  "delta_m_ref"
  w_PLL/1 -> Sum5/2
  Sum5/1 -> frequency/1, Sum6/2
  2*pi2/1 -> Sum1/3  "Control Delay Compensation"
  Integrator2/1 -> Sum1/2
  mp2/1 -> Switch/1
  2*pi3/1 -> Switch/2
  2*pi4/1 -> Switch/3

== system VSC_GFo_Variable_Frequency_v1/VSC00/Strategy 1/abc --> dq ==
  ig_abc : Inport
  Theta : Inport  Port=2
  Demux3 : Demux  Outputs=3
  Mux2 : Mux  Inputs=2
  abc_alpha_beta_tri4 : Subsystem
  abc_dq2 : Subsystem
  ig_dq_mes : Outport  VectorParamsAs1DForOutWhenUnconnected=off
  wires:
  Mux2/1 -> ig_dq_mes/1
  abc_alpha_beta_tri4/1(alpha) -> abc_dq2/2(a)
  Demux3/1 -> abc_alpha_beta_tri4/1(a)
  Demux3/2 -> abc_alpha_beta_tri4/2(b)
  abc_dq2/1(d) -> Mux2/1
  abc_alpha_beta_tri4/2(beta) -> abc_dq2/3(b)
  abc_dq2/2(q) -> Mux2/2
  ig_abc/1 -> Demux3/1
  Demux3/3 -> abc_alpha_beta_tri4/3(c)
  Theta/1 -> abc_dq2/1(Theta)

== system VSC_GFo_Variable_Frequency_v1/VSC00/Strategy 1/dq  -->  abc  ==
  Theta : Inport
  e_dq : Inport  Port=2
  Demux2 : Demux  Outputs=2
  Scope1 : Scope
  abc_alpha_beta : Subsystem
  abc_dq2 : Subsystem
  e_a_ref : Outport  VectorParamsAs1DForOutWhenUnconnected=off
  e_b_ref : Outport  Port=2  VectorParamsAs1DForOutWhenUnconnected=off
  e_c_ref : Outport  Port=3  VectorParamsAs1DForOutWhenUnconnected=off
  wires:
  abc_dq2/1(a) -> abc_alpha_beta/1(a)
  abc_dq2/2(b) -> abc_alpha_beta/2(b)
  Demux2/1 -> abc_dq2/2(d)
  Demux2/2 -> abc_dq2/3(q)
  Theta/1 -> abc_dq2/1(Theta)
  abc_alpha_beta/2(b1) -> e_b_ref/1
  e_dq/1 -> Demux2/1, Scope1/1
  abc_alpha_beta/3(c) -> e_c_ref/1
  abc_alpha_beta/1(a1) -> e_a_ref/1

== system VSC_GFo_Variable_Frequency_v1/VSC00/Strategy 2/ Active & Reactive Power ==
  e_abc : Inport  PortDimensions=3
  Ig_abc : Inport  Port=2  PortDimensions=3
  Demux : Demux  Outputs=3
  Mux : Mux  Inputs=3
  Product1 : Product  SaturateOnIntegerOverflow=on  InputSameDT=on  OutDataTypeStr=Inherit: Same as first input
  Product3 : Product  SaturateOnIntegerOverflow=on  InputSameDT=on  OutDataTypeStr=Inherit: Same as first input
  Sum : Sum  Inputs=+-  SaturateOnIntegerOverflow=on  InputSameDT=on  OutDataTypeStr=Inherit: Same as first input
  Sum1 : Sum  Inputs=1  SaturateOnIntegerOverflow=on  InputSameDT=on  OutDataTypeStr=Inherit: Same as first input
  Sum4 : Sum  Inputs=1  SaturateOnIntegerOverflow=on  InputSameDT=on  OutDataTypeStr=Inherit: Same as first input
  Sum5 : Sum  Inputs=+-  SaturateOnIntegerOverflow=on  InputSameDT=on  OutDataTypeStr=Inherit: Same as first input
  Sum6 : Sum  Inputs=+-  SaturateOnIntegerOverflow=on  InputSameDT=on  OutDataTypeStr=Inherit: Same as first input
  pu->V : Gain  Gain=1/sqrt(3)  SaturateOnIntegerOverflow=on  OutDataTypeStr=Inherit: Same as input  ParamDataTypeStr=Inherit: Same as input
  P : Outport  VectorParamsAs1DForOutWhenUnconnected=off
  Q : Outport  Port=2  VectorParamsAs1DForOutWhenUnconnected=off
  wires:
  pu->V/1 -> Q/1  "Q"
  Mux/1 -> Product3/1
  Sum6/1 -> Mux/2
  Sum5/1 -> Mux/1
  Sum/1 -> Mux/3
  Demux/3 -> Sum6/1, Sum5/2
  Demux/2 -> Sum5/1, Sum/2
  Demux/1 -> Sum6/2, Sum/1
  Sum4/1 -> P/1  "P"
  Ig_abc/1 -> Product3/2, Product1/2
  e_abc/1 -> Demux/1, Product1/1
  Product1/1 -> Sum4/1
  Product3/1 -> Sum1/1
  Sum1/1 -> pu->V/1

== system VSC_GFo_Variable_Frequency_v1/VSC00/Strategy 2/Damping ==
  i_gdq : Inport
  Filter w_LF : Subsystem
      mask Display: disp('\omega_{LF} / (s + \omega_{LF})','texmode','on')
  Sum5 : Sum  Inputs=|+-
  nq1 : Gain  Gain=Rv
  "D_Edq " : Outport  VectorParamsAs1DForOutWhenUnconnected=off
  wires:
  i_gdq/1 -> nq1/1
  Sum5/1 -> "D_Edq "/1
  Filter w_LF/1(s) -> Sum5/1
  nq1/1 -> Sum5/2, Filter w_LF/1(e)

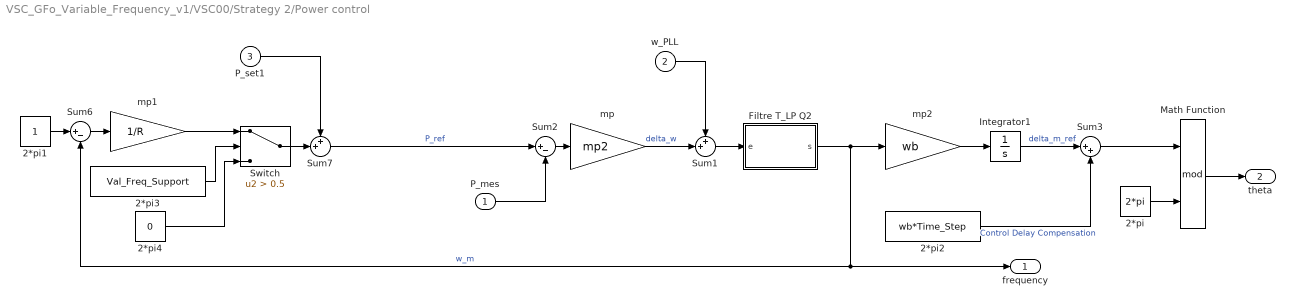
== system VSC_GFo_Variable_Frequency_v1/VSC00/Strategy 2/Power control ==
  P_mes : Inport
  w_PLL : Inport  Port=2
  P_set1 : Inport  Port=3
  2*pi : Constant  Value=2*pi
  2*pi1 : Constant
  2*pi2 : Constant  Value=wb*Time_Step
  2*pi3 : Constant  Value=Val_Freq_Support
  2*pi4 : Constant  Value=0
  Filtre T_LP Q2 : Subsystem
  Integrator1 : Integrator  InitialCondition=Theta_vsc0*pi/180
  Math Function : Math  Operator=mod  SaturateOnIntegerOverflow=on
  Sum1 : Sum  Inputs=++|
  Sum2 : Sum  Inputs=|+-
  Sum3 : Sum  Inputs=|++
  Sum6 : Sum  Inputs=|+-
  Sum7 : Sum  Inputs=++|
  Switch : Switch  Criteria=u2 > Threshold  Threshold=0.5
  mp : Gain  Gain=mp2
  mp1 : Gain  Gain=1/R
  mp2 : Gain  Gain=wb
  frequency : Outport  VectorParamsAs1DForOutWhenUnconnected=off
  theta : Outport  Port=2  VectorParamsAs1DForOutWhenUnconnected=off
  wires:
  Sum1/1 -> Filtre T_LP Q2/1(e)
  2*pi/1 -> Math Function/2
  Math Function/1 -> theta/1
  Integrator1/1 -> Sum3/1  "delta_m_ref"
  Sum2/1 -> mp/1
  mp/1 -> Sum1/2  "delta_w"
  Filtre T_LP Q2/1(s) -> mp2/1, frequency/1, Sum6/2  "w_m"
  w_PLL/1 -> Sum1/1
  P_mes/1 -> Sum2/2
  mp2/1 -> Integrator1/1
  2*pi2/1 -> Sum3/2  "Control Delay Compensation"
  Sum3/1 -> Math Function/1
  Switch/1 -> Sum7/2
  P_set1/1 -> Sum7/1
  Sum6/1 -> mp1/1
  2*pi1/1 -> Sum6/1
  mp1/1 -> Switch/1
  2*pi3/1 -> Switch/2
  2*pi4/1 -> Switch/3
  Sum7/1 -> Sum2/1  "P_ref"

== system VSC_GFo_Variable_Frequency_v1/VSC00/Strategy 2/abc --> dq ==
  ig_abc : Inport
  Theta : Inport  Port=2
  Demux3 : Demux  Outputs=3
  Mux2 : Mux  Inputs=2
  abc_alpha_beta_tri4 : Subsystem
  abc_dq2 : Subsystem
  ig_dq_mes : Outport  VectorParamsAs1DForOutWhenUnconnected=off
  wires:
  Mux2/1 -> ig_dq_mes/1
  abc_alpha_beta_tri4/1(alpha) -> abc_dq2/2(a)
  Demux3/1 -> abc_alpha_beta_tri4/1(a)
  Demux3/2 -> abc_alpha_beta_tri4/2(b)
  abc_dq2/1(d) -> Mux2/1
  abc_alpha_beta_tri4/2(beta) -> abc_dq2/3(b)
  abc_dq2/2(q) -> Mux2/2
  ig_abc/1 -> Demux3/1
  Demux3/3 -> abc_alpha_beta_tri4/3(c)
  Theta/1 -> abc_dq2/1(Theta)

== system VSC_GFo_Variable_Frequency_v1/VSC00/Strategy 2/dq  -->  abc  ==
  Theta : Inport
  e_dq : Inport  Port=2
  Demux2 : Demux  Outputs=2
  Scope1 : Scope
  abc_alpha_beta : Subsystem
  abc_dq2 : Subsystem
  e_a_ref : Outport  VectorParamsAs1DForOutWhenUnconnected=off
  e_b_ref : Outport  Port=2  VectorParamsAs1DForOutWhenUnconnected=off
  e_c_ref : Outport  Port=3  VectorParamsAs1DForOutWhenUnconnected=off
  wires:
  abc_dq2/1(a) -> abc_alpha_beta/1(a)
  abc_dq2/2(b) -> abc_alpha_beta/2(b)
  Demux2/1 -> abc_dq2/2(d)
  Demux2/2 -> abc_dq2/3(q)
  Theta/1 -> abc_dq2/1(Theta)
  abc_alpha_beta/2(b1) -> e_b_ref/1
  e_dq/1 -> Demux2/1, Scope1/1
  abc_alpha_beta/3(c) -> e_c_ref/1
  abc_alpha_beta/1(a1) -> e_a_ref/1

== system VSC_GFo_Variable_Frequency_v1/VSC00/Strategy 3/ Active & Reactive Power ==
  e_abc : Inport  PortDimensions=3
  Ig_abc : Inport  Port=2  PortDimensions=3
  Demux : Demux  Outputs=3
  Mux : Mux  Inputs=3
  Product1 : Product  SaturateOnIntegerOverflow=on  InputSameDT=on  OutDataTypeStr=Inherit: Same as first input
  Product3 : Product  SaturateOnIntegerOverflow=on  InputSameDT=on  OutDataTypeStr=Inherit: Same as first input
  Sum : Sum  Inputs=+-  SaturateOnIntegerOverflow=on  InputSameDT=on  OutDataTypeStr=Inherit: Same as first input
  Sum1 : Sum  Inputs=1  SaturateOnIntegerOverflow=on  InputSameDT=on  OutDataTypeStr=Inherit: Same as first input
  Sum4 : Sum  Inputs=1  SaturateOnIntegerOverflow=on  InputSameDT=on  OutDataTypeStr=Inherit: Same as first input
  Sum5 : Sum  Inputs=+-  SaturateOnIntegerOverflow=on  InputSameDT=on  OutDataTypeStr=Inherit: Same as first input
  Sum6 : Sum  Inputs=+-  SaturateOnIntegerOverflow=on  InputSameDT=on  OutDataTypeStr=Inherit: Same as first input
  pu->V : Gain  Gain=1/sqrt(3)  SaturateOnIntegerOverflow=on  OutDataTypeStr=Inherit: Same as input  ParamDataTypeStr=Inherit: Same as input
  P : Outport  VectorParamsAs1DForOutWhenUnconnected=off
  Q : Outport  Port=2  VectorParamsAs1DForOutWhenUnconnected=off
  wires:
  pu->V/1 -> Q/1  "Q"
  Mux/1 -> Product3/1
  Sum6/1 -> Mux/2
  Sum5/1 -> Mux/1
  Sum/1 -> Mux/3
  Demux/3 -> Sum6/1, Sum5/2
  Demux/2 -> Sum5/1, Sum/2
  Demux/1 -> Sum6/2, Sum/1
  Sum4/1 -> P/1  "P"
  Ig_abc/1 -> Product3/2, Product1/2
  e_abc/1 -> Demux/1, Product1/1
  Product1/1 -> Sum4/1
  Product3/1 -> Sum1/1
  Sum1/1 -> pu->V/1

== system VSC_GFo_Variable_Frequency_v1/VSC00/Strategy 3/Damping ==
  i_gdq : Inport
  Filter w_LF : Subsystem
      mask Display: disp('\omega_{LF} / (s + \omega_{LF})','texmode','on')
  Sum5 : Sum  Inputs=|+-
  nq1 : Gain  Gain=Rv
  "D_Edq " : Outport  VectorParamsAs1DForOutWhenUnconnected=off
  wires:
  i_gdq/1 -> nq1/1
  Sum5/1 -> "D_Edq "/1
  Filter w_LF/1(s) -> Sum5/1
  nq1/1 -> Sum5/2, Filter w_LF/1(e)
